simulink model "sgMdl_BMTS_FaultInsertionWithFIU"  (R2024b)
settings: Solver=FixedStepAuto  StartTime=0.0  StopTime=inf  RelTol=1e-3  EnableMultiTasking=on
undefined symbols (not defined in the file): Device_01, FIU12, FIU_12Ch_Set_init, sg_bce
libraries: slrealtimeethercatlib x27, simulink x13, SignalEditorBlockLib x1
Description:
  | BMTS - Fault Insertion with FIU
settings Model: ModifiedByFormat=Speedgoat  SimulationMode=external  ExtModeTrigDuration=100000  Creator=Speedgoat  LastModifiedBy=Speedgoat
settings SolverCC: ConcurrentTasks=on  AlgebraicLoopSolver=TrustRegion  PositivePriorityOrder=on  InsertRTBMode=Never (minimum delay)
settings DataIOCC: SaveFormat=Array  SaveState=on  SignalLoggingName=logsOut
settings OptimizationCC: BlockReduction=off  BooleanDataType=off  OptimizeBlockIOStorage=off  BufferReuse=off  ReuseModelBlockBuffer=off  GlobalBufferReuse=off  ExpressionFolding=off  LocalBlockOutputs=off  InitFltsAndDblsToZero=on  OptimizeDataStoreBuffers=off  BusAssignmentInplaceUpdate=off
settings DebuggingCC: SaveWithParameterizedLinksMsg=none  MergeDetectMultiDrivingBlocksExec=none  CheckExecutionContextPreStartOutputMsg=on  SignalResolutionControl=TryResolveAllWithWarning  TasksWithSamePriorityMsg=none  UnconnectedInputMsg=warning  UnconnectedOutputMsg=warning  UnconnectedLineMsg=warning  SFUnexpectedBacktrackingDiag=warning  SFNoUnconditionalDefaultTransitionDiag=warning  SFExecutionAtInitializationDiag=none  ArithmeticOperatorsInVariantConditions=warning
settings HardwareCC: ProdBitPerLong=64  ProdLongLongMode=on  ProdHWDeviceType=Intel->x86-64 (Linux 64)
settings ModelReferenceCC: EnableRefExpFcnMdlSchedulingChecks=on  PropagateSignalLabelsOutOfModel=off
settings SFSimCC: SimUseLocalCustomCode=off  SimTargetLang=C++
settings RTWCC: Description=Speedgoat Real-Time Target Machine  SystemTargetFile=speedgoat.tlc  TemplateMakefile=slrealtime_default_tmf  RTWUseLocalCustomCode=off  Toolchain=Simulink Real-Time Toolchain  BuildConfiguration=Faster Runs  TargetLang=C++  GPUComputeCapability=3.5  DLArmComputeVersion=19.05
settings CodeAppCC: StateflowObjectComments=on
settings SimulinkRealTimeTargetCC: SubcomponentCodeInterfacePackaging=Reusable function  InstructionSetFMA=off  LogToMDFFile=off  SLRTFileLogMaxRuns=10
settings ConfigComp: CovMetricSettings=dw  CovSaveCumulativeToWorkspaceVar=on  CovSaveSingleToWorkspaceVar=on  CovExternalEMLEnable=off  CovSFcnEnable=off  CovBoundaryAbsTol=1.0e-5

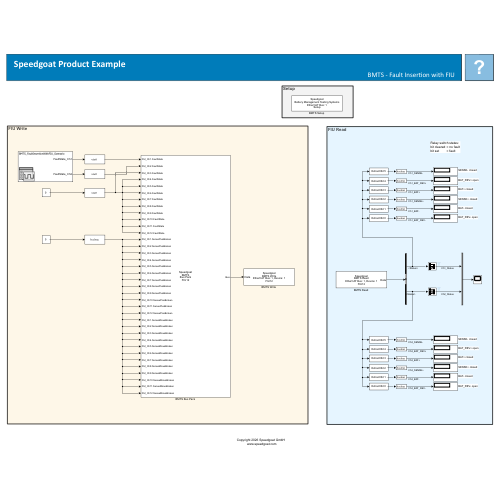
[thumbnail: Simulink's stored preview of the top-level diagram]
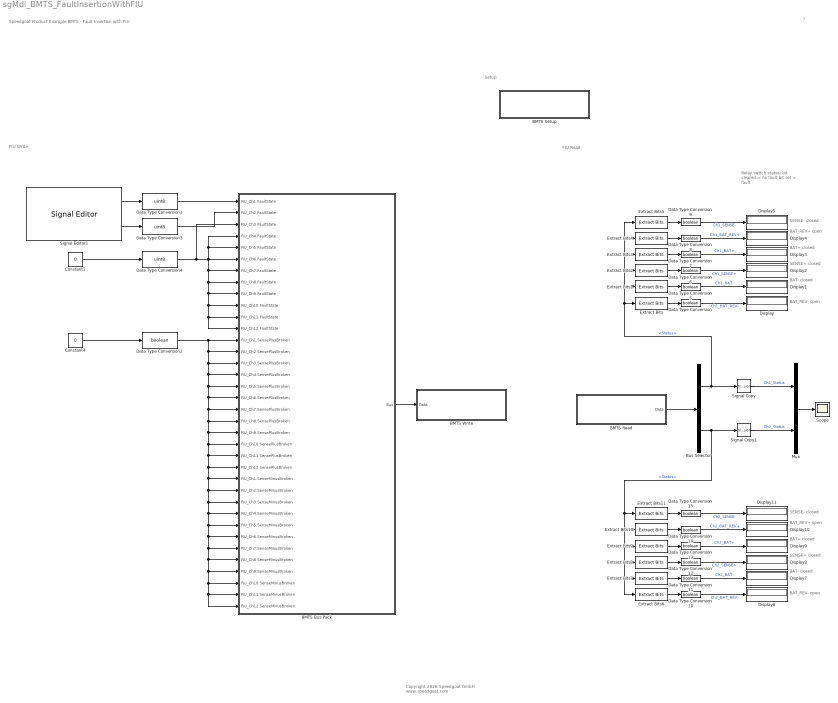
== system sgMdl_BMTS_FaultInsertionWithFIU ==
  note: BAT_REV- open
  note: Setup
  note: FIU Write
  note: FIU Read
  note: BAT- closed
  note: SENSE+ closed
  note: BAT+ closed
  note: BAT_REV+ open
  note: SENSE- closed
  note: Relay switch states:
      | bit cleared = no fault
      | bit set = fault
  note: BAT+ closed
  note: BAT_REV+ open
  note: BAT- closed
  note: SENSE+ closed
  note: BAT_REV- open
  note: SENSE- closed
  note: Speedgoat Product Example
      | BMTS - Fault Insertion with FIU
  note: ?
  note: Copyright 2026 Speedgoat GmbH
      |  www.speedgoat.com
  "BMTS Bus Pack " : Subsystem  mask(bmts_bus_pack){}
      settings: OpenFcn=sg_bce.openFcnBuspack;
      mask Help: eval('sg.utils.help.show(''io_main/refentry_bmts_buspack'');')
      mask Display: disp('Speedgoat\nBMTS\nBus Pack\nFIU12');
  "BMTS Read " : Subsystem  LoadFcn=sg_bce.createFiuTseBusSignals(12,0);  InitFcn=|  mask(bce_read){}
      | sg_bce.createFiuTseBusSignals(12,0);
      | sg_bce.checkNumberOfBlocksGlobal(bdroot);
      settings: OpenFcn=sg_bce.openFcnRead;
      mask Help: eval('sg.utils.help.show(''io_main/refentry_bce_read'');')
      mask Display: disp('Speedgoat\nBMTS Read\nEtherCAT Bus: 1, Device: 1\nFIU12');port_label('output',1,'Data');
  "BMTS Setup " : Subsystem  LoadFcn=|  InitFcn=|  mask(bce_setup){}
      LoadFcn=|
      | sg_bce.createBusSignals;
      | sg_bce.setupEniCallback(gcb, bdroot);
      InitFcn=|
      | sg_bce.createBusSignals;
      | sg_bce.checkNumberOfBlocksGlobal(bdroot);
      | sg_bce.setupEniCallback(gcb, bdroot);
      settings: OpenFcn=sg_bce.openFcnSetup;
      mask Help: eval('sg.utils.help.show(''io_main/refentry_bce_setup'');')
      mask Display: disp('Speedgoat\nBattery Management Testing Systems\nEtherCAT Bus: 1\nSetup');
  "BMTS Write " : Subsystem  LoadFcn=sg_bce.createFiuTseBusSignals(12,0);  InitFcn=|  mask(bce_write){}
      | sg_bce.createFiuTseBusSignals(12,0);
      | sg_bce.checkNumberOfBlocksGlobal(bdroot);
      settings: OpenFcn=sg_bce.openFcnWrite;
      mask Help: eval('sg.utils.help.show(''io_main/refentry_bce_write'');')
      mask Display: disp('Speedgoat\nBMTS Write\nEtherCAT Bus: 1, Device: 1\nFIU12');port_label('input',1,'Data');
  Bus Selector : BusSelector  OutputSignals=FIU_Ch1.Status,FIU_Ch2.Status
  Constant2 : Constant  Value=0
  Constant4 : Constant  Value=0
  Data Type Conversion{,2,5..15} (13 alike) : DataTypeConversion  OutDataTypeStr=boolean  SaturateOnIntegerOverflow=off  RndMeth=Floor
  Data Type Conversion1 : DataTypeConversion  OutDataTypeStr=uint8  SaturateOnIntegerOverflow=off  RndMeth=Floor
  Data Type Conversion3 : DataTypeConversion  OutDataTypeStr=uint8  SaturateOnIntegerOverflow=off  RndMeth=Floor
  Data Type Conversion4 : DataTypeConversion  OutDataTypeStr=uint8  SaturateOnIntegerOverflow=off  RndMeth=Floor
  Display{,1..11} (12 alike) : Display
  Extract Bits : simulink/Logic and Bit Operations/Extract Bits  bitsToExtract=Range of bits  numBits=8  bitIdxRange=[0]  outScalingMode=Treat bit field as an integer
  Extract Bits1 : simulink/Logic and Bit Operations/Extract Bits  bitsToExtract=Range of bits  numBits=8  bitIdxRange=[1]  outScalingMode=Treat bit field as an integer
  Extract Bits10 : simulink/Logic and Bit Operations/Extract Bits  bitsToExtract=Range of bits  numBits=8  bitIdxRange=[4]  outScalingMode=Treat bit field as an integer
  Extract Bits11 : simulink/Logic and Bit Operations/Extract Bits  bitsToExtract=Range of bits  numBits=8  bitIdxRange=[5]  outScalingMode=Treat bit field as an integer
  Extract Bits2 : simulink/Logic and Bit Operations/Extract Bits  bitsToExtract=Range of bits  numBits=8  bitIdxRange=[2]  outScalingMode=Treat bit field as an integer
  Extract Bits3 : simulink/Logic and Bit Operations/Extract Bits  bitsToExtract=Range of bits  numBits=8  bitIdxRange=[3]  outScalingMode=Treat bit field as an integer
  Extract Bits4 : simulink/Logic and Bit Operations/Extract Bits  bitsToExtract=Range of bits  numBits=8  bitIdxRange=[4]  outScalingMode=Treat bit field as an integer
  Extract Bits5 : simulink/Logic and Bit Operations/Extract Bits  bitsToExtract=Range of bits  numBits=8  bitIdxRange=[5]  outScalingMode=Treat bit field as an integer
  Extract Bits6 : simulink/Logic and Bit Operations/Extract Bits  bitsToExtract=Range of bits  numBits=8  bitIdxRange=[0]  outScalingMode=Treat bit field as an integer
  Extract Bits7 : simulink/Logic and Bit Operations/Extract Bits  bitsToExtract=Range of bits  numBits=8  bitIdxRange=[1]  outScalingMode=Treat bit field as an integer
  Extract Bits8 : simulink/Logic and Bit Operations/Extract Bits  bitsToExtract=Range of bits  numBits=8  bitIdxRange=[2]  outScalingMode=Treat bit field as an integer
  Extract Bits9 : simulink/Logic and Bit Operations/Extract Bits  bitsToExtract=Range of bits  numBits=8  bitIdxRange=[3]  outScalingMode=Treat bit field as an integer
  Mux : Mux  Inputs=2
  Scope : Scope
  Signal Copy : SignalConversion  OverrideOpt=off
  Signal Copy1 : SignalConversion  OverrideOpt=off
  Signal Editor1 : SignalEditorBlockLib/Signal Editor  FileName=BMTS_FaultInsertionWithFIU_Scenario.mat  ActiveScenario=BMTS_FaultInsertionWithFIU_Scenario  ActiveSignal=FaultState_Ch1  IsBus=off  OutputBusObjectStr=Bus: BusObject  SampleTime=0  Interpolate=off  ZeroCross=off  OutputAfterFinalValue=Setting to zero  Unit=inherit  PreserveSignalName=on  ApplySigPropsToAllScenarios=on  ApplySigPropsToAllSignals=off
  wires:
  "BMTS Read "/1(Data) -> Bus Selector/1
  Constant4/1 -> Data Type Conversion2/1
  Bus Selector/1 -> Extract Bits5/1, Extract Bits4/1, Extract Bits3/1, Extract Bits2/1, Extract Bits1/1, Extract Bits/1, Signal Copy/1  "<Status>"
  "BMTS Bus Pack "/1(Bus) -> "BMTS Write "/1(Data)
  Signal Editor1/1 -> Data Type Conversion1/1
  Data Type Conversion1/1 -> "BMTS Bus Pack "/1(FIU_Ch1.FaultState)
  Signal Editor1/2 -> Data Type Conversion3/1
  Data Type Conversion3/1 -> "BMTS Bus Pack "/2(FIU_Ch2.FaultState)
  Data Type Conversion2/1 -> "BMTS Bus Pack "/36(FIU_Ch12.SenseMinusBroken), "BMTS Bus Pack "/35(FIU_Ch11.SenseMinusBroken), "BMTS Bus Pack "/34(FIU_Ch10.SenseMinusBroken), "BMTS Bus Pack "/33(FIU_Ch9.SenseMinusBroken), "BMTS Bus Pack "/32(FIU_Ch8.SenseMinusBroken), "BMTS Bus Pack "/31(FIU_Ch7.SenseMinusBroken), "BMTS Bus Pack "/30(FIU_Ch6.SenseMinusBroken), "BMTS Bus Pack "/29(FIU_Ch5.SenseMinusBroken), "BMTS Bus Pack "/28(FIU_Ch4.SenseMinusBroken), "BMTS Bus Pack "/27(FIU_Ch3.SenseMinusBroken), "BMTS Bus Pack "/26(FIU_Ch2.SenseMinusBroken), "BMTS Bus Pack "/25(FIU_Ch1.SenseMinusBroken), "BMTS Bus Pack "/24(FIU_Ch12.SensePlusBroken), "BMTS Bus Pack "/23(FIU_Ch11.SensePlusBroken), "BMTS Bus Pack "/22(FIU_Ch10.SensePlusBroken), "BMTS Bus Pack "/21(FIU_Ch9.SensePlusBroken), "BMTS Bus Pack "/20(FIU_Ch8.SensePlusBroken), "BMTS Bus Pack "/19(FIU_Ch7.SensePlusBroken), "BMTS Bus Pack "/18(FIU_Ch6.SensePlusBroken), "BMTS Bus Pack "/17(FIU_Ch5.SensePlusBroken), "BMTS Bus Pack "/16(FIU_Ch4.SensePlusBroken), "BMTS Bus Pack "/15(FIU_Ch3.SensePlusBroken), "BMTS Bus Pack "/14(FIU_Ch2.SensePlusBroken), "BMTS Bus Pack "/13(FIU_Ch1.SensePlusBroken)
  Constant2/1 -> Data Type Conversion4/1
  Data Type Conversion4/1 -> "BMTS Bus Pack "/11(FIU_Ch11.FaultState), "BMTS Bus Pack "/12(FIU_Ch12.FaultState), "BMTS Bus Pack "/10(FIU_Ch10.FaultState), "BMTS Bus Pack "/9(FIU_Ch9.FaultState), "BMTS Bus Pack "/8(FIU_Ch8.FaultState), "BMTS Bus Pack "/7(FIU_Ch7.FaultState), "BMTS Bus Pack "/4(FIU_Ch4.FaultState), "BMTS Bus Pack "/5(FIU_Ch5.FaultState), "BMTS Bus Pack "/6(FIU_Ch6.FaultState), "BMTS Bus Pack "/3(FIU_Ch3.FaultState)
  Mux/1 -> Scope/1
  Extract Bits/1 -> Data Type Conversion/1
  Extract Bits1/1 -> Data Type Conversion5/1
  Extract Bits2/1 -> Data Type Conversion6/1
  Extract Bits5/1 -> Data Type Conversion9/1
  Extract Bits4/1 -> Data Type Conversion8/1
  Extract Bits3/1 -> Data Type Conversion7/1
  Extract Bits9/1 -> Data Type Conversion13/1
  Extract Bits10/1 -> Data Type Conversion14/1
  Extract Bits11/1 -> Data Type Conversion15/1
  Extract Bits8/1 -> Data Type Conversion12/1
  Extract Bits7/1 -> Data Type Conversion11/1
  Extract Bits6/1 -> Data Type Conversion10/1
  Bus Selector/2 -> Extract Bits6/1, Extract Bits7/1, Extract Bits8/1, Extract Bits9/1, Extract Bits10/1, Extract Bits11/1, Signal Copy1/1  "<Status>"
  Signal Copy/1 -> Mux/1  "Ch1_Status"
  Signal Copy1/1 -> Mux/2  "Ch2_Status"
  Data Type Conversion/1 -> Display/1  "Ch1_BAT_REV-"
  Data Type Conversion5/1 -> Display1/1  "Ch1_BAT-"
  Data Type Conversion6/1 -> Display2/1  "Ch1_SENSE+"
  Data Type Conversion7/1 -> Display3/1  "Ch1_BAT+"
  Data Type Conversion8/1 -> Display4/1  "Ch1_BAT_REV+"
  Data Type Conversion9/1 -> Display5/1  "Ch1_SENSE-"
  Data Type Conversion12/1 -> Display8/1  "Ch2_SENSE+"
  Data Type Conversion10/1 -> Display6/1  "Ch2_BAT_REV-"
  Data Type Conversion14/1 -> Display10/1  "Ch2_BAT_REV+"
  Data Type Conversion15/1 -> Display11/1  "Ch2_SENSE-"
  Data Type Conversion11/1 -> Display7/1  "Ch2_BAT-"
  Data Type Conversion13/1 -> Display9/1  "Ch2_BAT+"

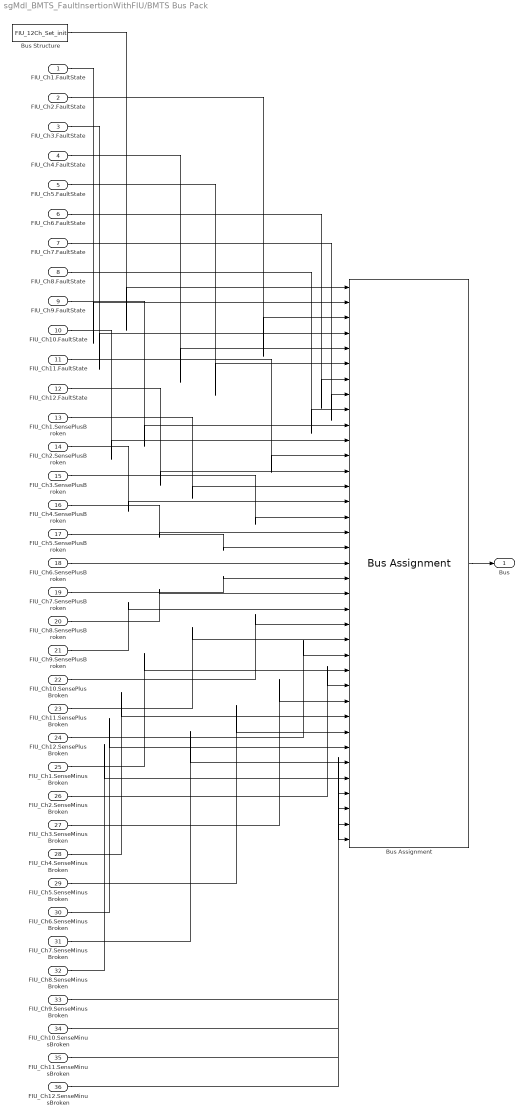
== system sgMdl_BMTS_FaultInsertionWithFIU/BMTS Bus Pack  ==
  FIU_Ch1.FaultState : Inport
  FIU_Ch2.FaultState : Inport  Port=2
  FIU_Ch3.FaultState : Inport  Port=3
  FIU_Ch4.FaultState : Inport  Port=4
  FIU_Ch5.FaultState : Inport  Port=5
  FIU_Ch6.FaultState : Inport  Port=6
  FIU_Ch7.FaultState : Inport  Port=7
  FIU_Ch8.FaultState : Inport  Port=8
  FIU_Ch9.FaultState : Inport  Port=9
  FIU_Ch10.FaultState : Inport  Port=10
  FIU_Ch11.FaultState : Inport  Port=11
  FIU_Ch12.FaultState : Inport  Port=12
  FIU_Ch1.SensePlusBroken : Inport  Port=13
  FIU_Ch2.SensePlusBroken : Inport  Port=14
  FIU_Ch3.SensePlusBroken : Inport  Port=15
  FIU_Ch4.SensePlusBroken : Inport  Port=16
  FIU_Ch5.SensePlusBroken : Inport  Port=17
  FIU_Ch6.SensePlusBroken : Inport  Port=18
  FIU_Ch7.SensePlusBroken : Inport  Port=19
  FIU_Ch8.SensePlusBroken : Inport  Port=20
  FIU_Ch9.SensePlusBroken : Inport  Port=21
  FIU_Ch10.SensePlusBroken : Inport  Port=22
  FIU_Ch11.SensePlusBroken : Inport  Port=23
  FIU_Ch12.SensePlusBroken : Inport  Port=24
  FIU_Ch1.SenseMinusBroken : Inport  Port=25
  FIU_Ch2.SenseMinusBroken : Inport  Port=26
  FIU_Ch3.SenseMinusBroken : Inport  Port=27
  FIU_Ch4.SenseMinusBroken : Inport  Port=28
  FIU_Ch5.SenseMinusBroken : Inport  Port=29
  FIU_Ch6.SenseMinusBroken : Inport  Port=30
  FIU_Ch7.SenseMinusBroken : Inport  Port=31
  FIU_Ch8.SenseMinusBroken : Inport  Port=32
  FIU_Ch9.SenseMinusBroken : Inport  Port=33
  FIU_Ch10.SenseMinusBroken : Inport  Port=34
  FIU_Ch11.SenseMinusBroken : Inport  Port=35
  FIU_Ch12.SenseMinusBroken : Inport  Port=36
  Bus Assignment : BusAssignment  AssignedSignals=FIU_Ch1.FaultState,FIU_Ch2.FaultState,FIU_Ch3.FaultState,FIU_Ch4.FaultState,FIU_Ch5.FaultState,FIU_Ch6.FaultState,FIU_Ch7.FaultState,FIU_Ch8.FaultState,FIU_Ch9.FaultState,FIU_Ch10.FaultState,FIU_Ch11.FaultState,FIU_Ch12.FaultState,FIU_Ch1.SensePlusBroken,FIU_Ch2.SensePlusBroken,FIU_Ch3.SensePlusBroken,FIU_Ch4.SensePlusBroken,FIU_Ch5.SensePlusBroken,FIU_Ch6.SensePlusBroken,FIU_Ch7.SensePlusBroken,FIU_Ch8.SensePlusBroken,FIU_Ch9.SensePlusBroken,FIU_Ch10.SensePlusBroken,FIU_Ch11.SensePlusBroken,FIU_Ch12.SensePlusBroken,FIU_Ch1.SenseMinusBroken,FIU_Ch2.SenseMinusBroken,FIU_Ch3.SenseMinusBroken,FIU_Ch4.SenseMinusBroken,FIU_Ch5.SenseMinusBroken,FIU_Ch6.SenseMinusBroken,FIU_Ch7.SenseMinusBroken,FIU_Ch8.SenseMinusBroken,FIU_Ch9.SenseMinusBroken,FIU_Ch10.SenseMinusBroken,FIU_Ch11.SenseMinusBroken,FIU_Ch12.SenseMinusBroken
  Bus Structure : Constant  Value=FIU_12Ch_Set_init  OutDataTypeStr=Bus: FIU_12Ch_Set
  Bus : Outport
  wires:
  Bus Structure/1 -> Bus Assignment/1
  FIU_Ch5.SenseMinusBroken/1 -> Bus Assignment/30
  FIU_Ch1.FaultState/1 -> Bus Assignment/2
  FIU_Ch2.FaultState/1 -> Bus Assignment/3
  FIU_Ch7.SenseMinusBroken/1 -> Bus Assignment/32
  FIU_Ch3.FaultState/1 -> Bus Assignment/4
  FIU_Ch5.FaultState/1 -> Bus Assignment/6
  FIU_Ch4.FaultState/1 -> Bus Assignment/5
  FIU_Ch2.SensePlusBroken/1 -> Bus Assignment/15
  FIU_Ch7.FaultState/1 -> Bus Assignment/8
  FIU_Ch8.SensePlusBroken/1 -> Bus Assignment/21
  FIU_Ch3.SensePlusBroken/1 -> Bus Assignment/16
  FIU_Ch8.FaultState/1 -> Bus Assignment/9
  FIU_Ch6.FaultState/1 -> Bus Assignment/7
  FIU_Ch7.SensePlusBroken/1 -> Bus Assignment/20
  FIU_Ch9.FaultState/1 -> Bus Assignment/10
  FIU_Ch10.FaultState/1 -> Bus Assignment/11
  FIU_Ch11.FaultState/1 -> Bus Assignment/12
  FIU_Ch12.FaultState/1 -> Bus Assignment/13
  FIU_Ch5.SensePlusBroken/1 -> Bus Assignment/18
  FIU_Ch1.SensePlusBroken/1 -> Bus Assignment/14
  FIU_Ch4.SensePlusBroken/1 -> Bus Assignment/17
  FIU_Ch2.SenseMinusBroken/1 -> Bus Assignment/27
  FIU_Ch6.SensePlusBroken/1 -> Bus Assignment/19
  FIU_Ch9.SensePlusBroken/1 -> Bus Assignment/22
  FIU_Ch10.SensePlusBroken/1 -> Bus Assignment/23
  FIU_Ch11.SensePlusBroken/1 -> Bus Assignment/24
  FIU_Ch12.SensePlusBroken/1 -> Bus Assignment/25
  FIU_Ch1.SenseMinusBroken/1 -> Bus Assignment/26
  FIU_Ch3.SenseMinusBroken/1 -> Bus Assignment/28
  FIU_Ch6.SenseMinusBroken/1 -> Bus Assignment/31
  FIU_Ch4.SenseMinusBroken/1 -> Bus Assignment/29
  FIU_Ch8.SenseMinusBroken/1 -> Bus Assignment/33
  FIU_Ch9.SenseMinusBroken/1 -> Bus Assignment/34
  FIU_Ch10.SenseMinusBroken/1 -> Bus Assignment/35
  FIU_Ch11.SenseMinusBroken/1 -> Bus Assignment/36
  FIU_Ch12.SenseMinusBroken/1 -> Bus Assignment/37
  Bus Assignment/1 -> Bus/1

== system sgMdl_BMTS_FaultInsertionWithFIU/BMTS Read  ==
  Subsystem : Subsystem
  Data : Outport  OutDataTypeStr=Bus: FIU_12Ch_Get
  wires:
  Subsystem/1(Data) -> Data/1

== system sgMdl_BMTS_FaultInsertionWithFIU/BMTS Setup  ==
  EtherCAT Init : slrealtimeethercatlib/EtherCAT Init  Priority=0  config_file=C:\Users\timo.straessle\AppData\Local\Temp\sg_bmts\sgMdl_BMTS_FaultInsertionWithFIU\sg_bmts_ENI_bus1.xml  device_id=1  portnum=1  initstate=2  dctuning=0  enaDebug=0  logFile='c:\dbglog.txt'  sample_time=0.001000  DCMode=0
  Terminator : Terminator
  wires:
  EtherCAT Init/1 -> Terminator/1

== system sgMdl_BMTS_FaultInsertionWithFIU/BMTS Write  ==
  Data : Inport  OutDataTypeStr=Bus: FIU_12Ch_Set
  Subsystem : Subsystem
  wires:
  Data/1 -> Subsystem/1(Data)

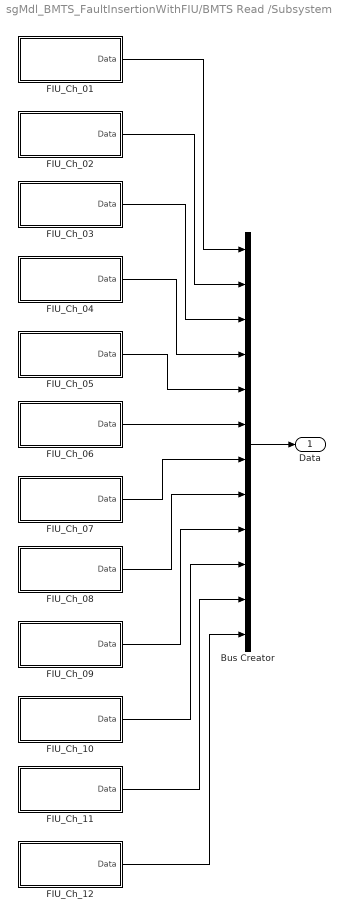
== system sgMdl_BMTS_FaultInsertionWithFIU/BMTS Read /Subsystem ==
  Bus Creator : BusCreator  Inputs=12  OutDataTypeStr=Bus: FIU_12Ch_Get
      settings: InheritFromInputs=off
  FIU_Ch_01 : Subsystem
  FIU_Ch_02 : Subsystem
  FIU_Ch_03 : Subsystem
  FIU_Ch_04 : Subsystem
  FIU_Ch_05 : Subsystem
  FIU_Ch_06 : Subsystem
  FIU_Ch_07 : Subsystem
  FIU_Ch_08 : Subsystem
  FIU_Ch_09 : Subsystem
  FIU_Ch_10 : Subsystem
  FIU_Ch_11 : Subsystem
  FIU_Ch_12 : Subsystem
  Data : Outport  OutDataTypeStr=Bus: FIU_12Ch_Get
  wires:
  FIU_Ch_05/1(Data) -> Bus Creator/5
  FIU_Ch_03/1(Data) -> Bus Creator/3
  FIU_Ch_01/1(Data) -> Bus Creator/1
  FIU_Ch_04/1(Data) -> Bus Creator/4
  FIU_Ch_02/1(Data) -> Bus Creator/2
  FIU_Ch_08/1(Data) -> Bus Creator/8
  FIU_Ch_06/1(Data) -> Bus Creator/6
  FIU_Ch_07/1(Data) -> Bus Creator/7
  FIU_Ch_09/1(Data) -> Bus Creator/9
  FIU_Ch_10/1(Data) -> Bus Creator/10
  FIU_Ch_11/1(Data) -> Bus Creator/11
  FIU_Ch_12/1(Data) -> Bus Creator/12
  Bus Creator/1 -> Data/1

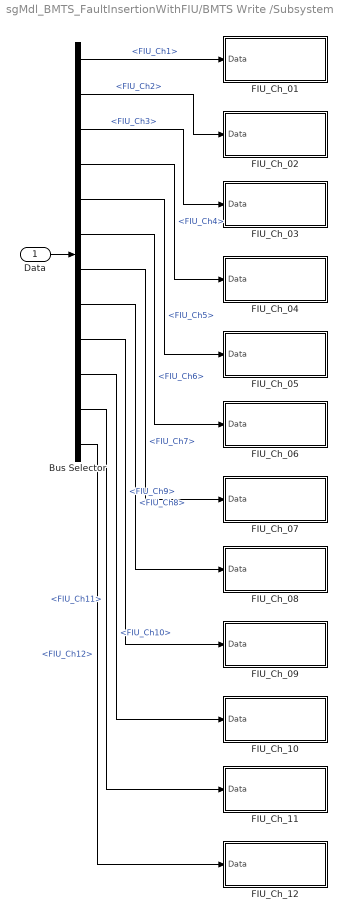
== system sgMdl_BMTS_FaultInsertionWithFIU/BMTS Write /Subsystem ==
  Data : Inport  OutDataTypeStr=Bus: FIU_12Ch_Set
  Bus Selector : BusSelector  OutputSignals=FIU_Ch1,FIU_Ch2,FIU_Ch3,FIU_Ch4,FIU_Ch5,FIU_Ch6,FIU_Ch7,FIU_Ch8,FIU_Ch9,FIU_Ch10,FIU_Ch11,FIU_Ch12
  FIU_Ch_01 : Subsystem
  FIU_Ch_02 : Subsystem
  FIU_Ch_03 : Subsystem
  FIU_Ch_04 : Subsystem
  FIU_Ch_05 : Subsystem
  FIU_Ch_06 : Subsystem
  FIU_Ch_07 : Subsystem
  FIU_Ch_08 : Subsystem
  FIU_Ch_09 : Subsystem
  FIU_Ch_10 : Subsystem
  FIU_Ch_11 : Subsystem
  FIU_Ch_12 : Subsystem
  wires:
  Data/1 -> Bus Selector/1
  Bus Selector/7 -> FIU_Ch_07/1(Data)  "<FIU_Ch7>"
  Bus Selector/6 -> FIU_Ch_06/1(Data)  "<FIU_Ch6>"
  Bus Selector/4 -> FIU_Ch_04/1(Data)  "<FIU_Ch4>"
  Bus Selector/3 -> FIU_Ch_03/1(Data)  "<FIU_Ch3>"
  Bus Selector/2 -> FIU_Ch_02/1(Data)  "<FIU_Ch2>"
  Bus Selector/1 -> FIU_Ch_01/1(Data)  "<FIU_Ch1>"
  Bus Selector/5 -> FIU_Ch_05/1(Data)  "<FIU_Ch5>"
  Bus Selector/8 -> FIU_Ch_08/1(Data)  "<FIU_Ch8>"
  Bus Selector/9 -> FIU_Ch_09/1(Data)  "<FIU_Ch9>"
  Bus Selector/10 -> FIU_Ch_10/1(Data)  "<FIU_Ch10>"
  Bus Selector/11 -> FIU_Ch_11/1(Data)  "<FIU_Ch11>"
  Bus Selector/12 -> FIU_Ch_12/1(Data)  "<FIU_Ch12>"

== system sgMdl_BMTS_FaultInsertionWithFIU/BMTS Read /Subsystem/FIU_Ch_01 ==
  note: Channel X
  Bus Creator : BusCreator  Inputs=1  OutDataTypeStr=Bus: FIU_Get
      settings: InheritFromInputs=off
  EtherCAT PDO Receive01 : slrealtimeethercatlib/EtherCAT PDO Receive  Priority=2  sig_name=Device_01 (FIU12).Tx_Channel_01.status  sig_offset=0  sig_type=uint8  type_size=8  sig_dim=1  device_id=1  sample_time=0.001000
  Data : Outport  OutDataTypeStr=Bus: FIU_Get
  wires:
  Bus Creator/1 -> Data/1
  EtherCAT PDO Receive01/1 -> Bus Creator/1  "ChX_Status"

== system sgMdl_BMTS_FaultInsertionWithFIU/BMTS Read /Subsystem/FIU_Ch_02 ==
  note: Channel X
  Bus Creator : BusCreator  Inputs=1  OutDataTypeStr=Bus: FIU_Get
      settings: InheritFromInputs=off
  EtherCAT PDO Receive01 : slrealtimeethercatlib/EtherCAT PDO Receive  Priority=2  sig_name=Device_01 (FIU12).Tx_Channel_02.status  sig_offset=8  sig_type=uint8  type_size=8  sig_dim=1  device_id=1  sample_time=0.001000
  Data : Outport  OutDataTypeStr=Bus: FIU_Get
  wires:
  Bus Creator/1 -> Data/1
  EtherCAT PDO Receive01/1 -> Bus Creator/1  "ChX_Status"

== system sgMdl_BMTS_FaultInsertionWithFIU/BMTS Read /Subsystem/FIU_Ch_03 ==
  note: Channel X
  Bus Creator : BusCreator  Inputs=1  OutDataTypeStr=Bus: FIU_Get
      settings: InheritFromInputs=off
  EtherCAT PDO Receive01 : slrealtimeethercatlib/EtherCAT PDO Receive  Priority=2  sig_name=Device_01 (FIU12).Tx_Channel_03.status  sig_offset=16  sig_type=uint8  type_size=8  sig_dim=1  device_id=1  sample_time=0.001000
  Data : Outport  OutDataTypeStr=Bus: FIU_Get
  wires:
  Bus Creator/1 -> Data/1
  EtherCAT PDO Receive01/1 -> Bus Creator/1  "ChX_Status"

== system sgMdl_BMTS_FaultInsertionWithFIU/BMTS Read /Subsystem/FIU_Ch_04 ==
  note: Channel X
  Bus Creator : BusCreator  Inputs=1  OutDataTypeStr=Bus: FIU_Get
      settings: InheritFromInputs=off
  EtherCAT PDO Receive01 : slrealtimeethercatlib/EtherCAT PDO Receive  Priority=2  sig_name=Device_01 (FIU12).Tx_Channel_04.status  sig_offset=24  sig_type=uint8  type_size=8  sig_dim=1  device_id=1  sample_time=0.001000
  Data : Outport  OutDataTypeStr=Bus: FIU_Get
  wires:
  Bus Creator/1 -> Data/1
  EtherCAT PDO Receive01/1 -> Bus Creator/1  "ChX_Status"

== system sgMdl_BMTS_FaultInsertionWithFIU/BMTS Read /Subsystem/FIU_Ch_05 ==
  note: Channel X
  Bus Creator : BusCreator  Inputs=1  OutDataTypeStr=Bus: FIU_Get
      settings: InheritFromInputs=off
  EtherCAT PDO Receive01 : slrealtimeethercatlib/EtherCAT PDO Receive  Priority=2  sig_name=Device_01 (FIU12).Tx_Channel_05.status  sig_offset=32  sig_type=uint8  type_size=8  sig_dim=1  device_id=1  sample_time=0.001000
  Data : Outport  OutDataTypeStr=Bus: FIU_Get
  wires:
  Bus Creator/1 -> Data/1
  EtherCAT PDO Receive01/1 -> Bus Creator/1  "ChX_Status"

== system sgMdl_BMTS_FaultInsertionWithFIU/BMTS Read /Subsystem/FIU_Ch_06 ==
  note: Channel X
  Bus Creator : BusCreator  Inputs=1  OutDataTypeStr=Bus: FIU_Get
      settings: InheritFromInputs=off
  EtherCAT PDO Receive01 : slrealtimeethercatlib/EtherCAT PDO Receive  Priority=2  sig_name=Device_01 (FIU12).Tx_Channel_06.status  sig_offset=40  sig_type=uint8  type_size=8  sig_dim=1  device_id=1  sample_time=0.001000
  Data : Outport  OutDataTypeStr=Bus: FIU_Get
  wires:
  Bus Creator/1 -> Data/1
  EtherCAT PDO Receive01/1 -> Bus Creator/1  "ChX_Status"

== system sgMdl_BMTS_FaultInsertionWithFIU/BMTS Read /Subsystem/FIU_Ch_07 ==
  note: Channel X
  Bus Creator : BusCreator  Inputs=1  OutDataTypeStr=Bus: FIU_Get
      settings: InheritFromInputs=off
  EtherCAT PDO Receive01 : slrealtimeethercatlib/EtherCAT PDO Receive  Priority=2  sig_name=Device_01 (FIU12).Tx_Channel_07.status  sig_offset=48  sig_type=uint8  type_size=8  sig_dim=1  device_id=1  sample_time=0.001000
  Data : Outport  OutDataTypeStr=Bus: FIU_Get
  wires:
  Bus Creator/1 -> Data/1
  EtherCAT PDO Receive01/1 -> Bus Creator/1  "ChX_Status"

== system sgMdl_BMTS_FaultInsertionWithFIU/BMTS Read /Subsystem/FIU_Ch_08 ==
  note: Channel X
  Bus Creator : BusCreator  Inputs=1  OutDataTypeStr=Bus: FIU_Get
      settings: InheritFromInputs=off
  EtherCAT PDO Receive01 : slrealtimeethercatlib/EtherCAT PDO Receive  Priority=2  sig_name=Device_01 (FIU12).Tx_Channel_08.status  sig_offset=56  sig_type=uint8  type_size=8  sig_dim=1  device_id=1  sample_time=0.001000
  Data : Outport  OutDataTypeStr=Bus: FIU_Get
  wires:
  Bus Creator/1 -> Data/1
  EtherCAT PDO Receive01/1 -> Bus Creator/1  "ChX_Status"

== system sgMdl_BMTS_FaultInsertionWithFIU/BMTS Read /Subsystem/FIU_Ch_09 ==
  note: Channel X
  Bus Creator : BusCreator  Inputs=1  OutDataTypeStr=Bus: FIU_Get
      settings: InheritFromInputs=off
  EtherCAT PDO Receive01 : slrealtimeethercatlib/EtherCAT PDO Receive  Priority=2  sig_name=Device_01 (FIU12).Tx_Channel_09.status  sig_offset=64  sig_type=uint8  type_size=8  sig_dim=1  device_id=1  sample_time=0.001000
  Data : Outport  OutDataTypeStr=Bus: FIU_Get
  wires:
  Bus Creator/1 -> Data/1
  EtherCAT PDO Receive01/1 -> Bus Creator/1  "ChX_Status"

== system sgMdl_BMTS_FaultInsertionWithFIU/BMTS Read /Subsystem/FIU_Ch_10 ==
  note: Channel X
  Bus Creator : BusCreator  Inputs=1  OutDataTypeStr=Bus: FIU_Get
      settings: InheritFromInputs=off
  EtherCAT PDO Receive01 : slrealtimeethercatlib/EtherCAT PDO Receive  Priority=2  sig_name=Device_01 (FIU12).Tx_Channel_10.status  sig_offset=72  sig_type=uint8  type_size=8  sig_dim=1  device_id=1  sample_time=0.001000
  Data : Outport  OutDataTypeStr=Bus: FIU_Get
  wires:
  Bus Creator/1 -> Data/1
  EtherCAT PDO Receive01/1 -> Bus Creator/1  "ChX_Status"

== system sgMdl_BMTS_FaultInsertionWithFIU/BMTS Read /Subsystem/FIU_Ch_11 ==
  note: Channel X
  Bus Creator : BusCreator  Inputs=1  OutDataTypeStr=Bus: FIU_Get
      settings: InheritFromInputs=off
  EtherCAT PDO Receive01 : slrealtimeethercatlib/EtherCAT PDO Receive  Priority=2  sig_name=Device_01 (FIU12).Tx_Channel_11.status  sig_offset=80  sig_type=uint8  type_size=8  sig_dim=1  device_id=1  sample_time=0.001000
  Data : Outport  OutDataTypeStr=Bus: FIU_Get
  wires:
  Bus Creator/1 -> Data/1
  EtherCAT PDO Receive01/1 -> Bus Creator/1  "ChX_Status"

== system sgMdl_BMTS_FaultInsertionWithFIU/BMTS Read /Subsystem/FIU_Ch_12 ==
  note: Channel X
  Bus Creator : BusCreator  Inputs=1  OutDataTypeStr=Bus: FIU_Get
      settings: InheritFromInputs=off
  EtherCAT PDO Receive01 : slrealtimeethercatlib/EtherCAT PDO Receive  Priority=2  sig_name=Device_01 (FIU12).Tx_Channel_12.status  sig_offset=88  sig_type=uint8  type_size=8  sig_dim=1  device_id=1  sample_time=0.001000
  Data : Outport  OutDataTypeStr=Bus: FIU_Get
  wires:
  Bus Creator/1 -> Data/1
  EtherCAT PDO Receive01/1 -> Bus Creator/1  "ChX_Status"

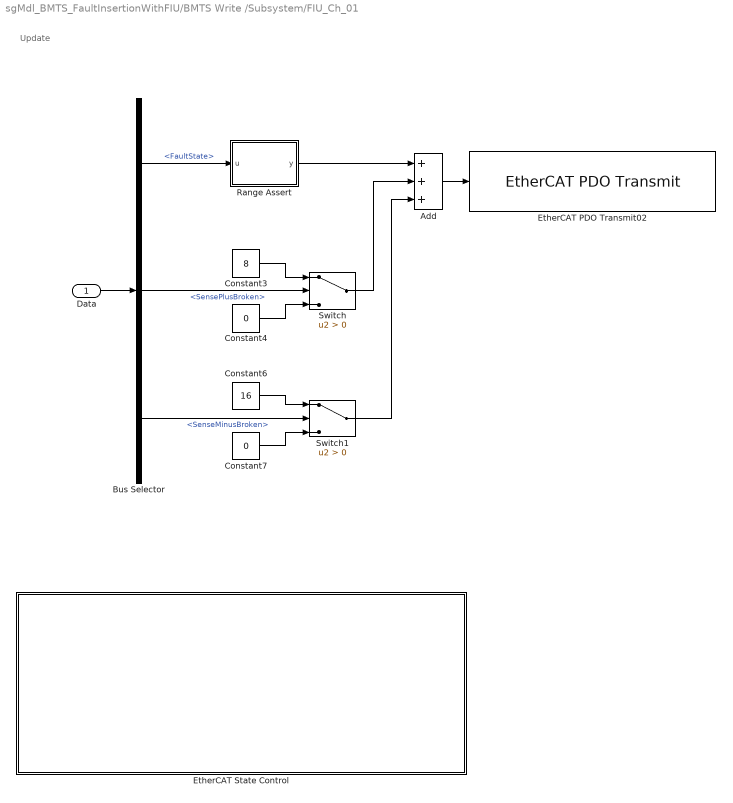
== system sgMdl_BMTS_FaultInsertionWithFIU/BMTS Write /Subsystem/FIU_Ch_01 ==
  note: Update
  Data : Inport  OutDataTypeStr=Bus: FIU_Set
  Add : Sum  Inputs=+++
  Bus Selector : BusSelector  OutputSignals=FaultState,SensePlusBroken,SenseMinusBroken
  Constant3 : Constant  Value=8  OutDataTypeStr=uint8
  Constant4 : Constant  Value=0  OutDataTypeStr=uint8
  Constant6 : Constant  Value=16  OutDataTypeStr=uint8
  Constant7 : Constant  Value=0  OutDataTypeStr=uint8
  EtherCAT PDO Transmit02 : slrealtimeethercatlib/EtherCAT PDO Transmit  Priority=3  sig_name=Device_01 (FIU12).Rx_Channel_01.faultState  sig_offset=0  sig_type=uint8  type_size=8  sig_dim=1  device_id=1  sample_time=0.001000
  EtherCAT State Control : Subsystem
  Range Assert : MATLAB Function  TreatAsAtomicUnit=on
  Switch : Switch  Criteria=u2 > Threshold  SaturateOnIntegerOverflow=off  InputSameDT=off
  Switch1 : Switch  Criteria=u2 > Threshold  SaturateOnIntegerOverflow=off  InputSameDT=off
  wires:
  Range Assert/1(y) -> Add/1
  Data/1 -> Bus Selector/1
  Bus Selector/2 -> Switch/2  "<SensePlusBroken>"
  Constant6/1 -> Switch1/1
  Constant3/1 -> Switch/1
  Switch/1 -> Add/2
  Constant4/1 -> Switch/3
  Constant7/1 -> Switch1/3
  Add/1 -> EtherCAT PDO Transmit02/1
  Bus Selector/3 -> Switch1/2  "<SenseMinusBroken>"
  Switch1/1 -> Add/3
  Bus Selector/1 -> Range Assert/1(u)  "<FaultState>"

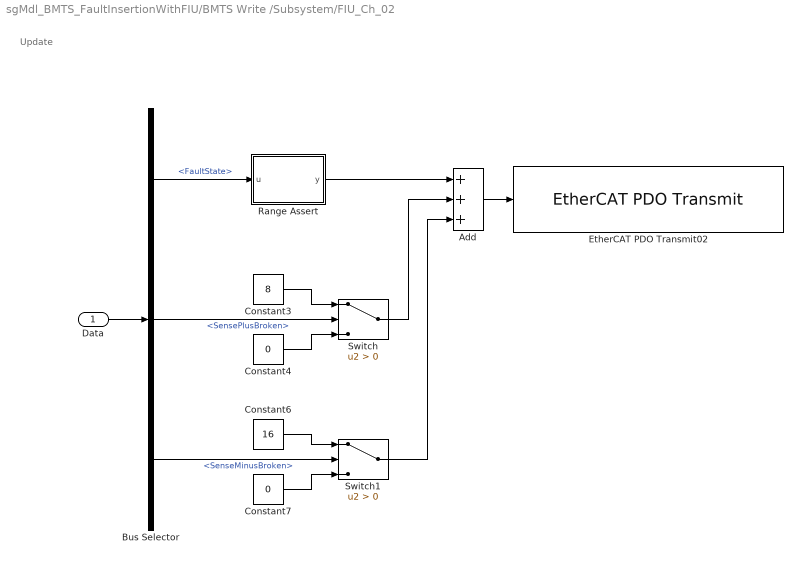
== system sgMdl_BMTS_FaultInsertionWithFIU/BMTS Write /Subsystem/FIU_Ch_02 ==
  note: Update
  Data : Inport  OutDataTypeStr=Bus: FIU_Set
  Add : Sum  Inputs=+++
  Bus Selector : BusSelector  OutputSignals=FaultState,SensePlusBroken,SenseMinusBroken
  Constant3 : Constant  Value=8  OutDataTypeStr=uint8
  Constant4 : Constant  Value=0  OutDataTypeStr=uint8
  Constant6 : Constant  Value=16  OutDataTypeStr=uint8
  Constant7 : Constant  Value=0  OutDataTypeStr=uint8
  EtherCAT PDO Transmit02 : slrealtimeethercatlib/EtherCAT PDO Transmit  Priority=3  sig_name=Device_01 (FIU12).Rx_Channel_02.faultState  sig_offset=8  sig_type=uint8  type_size=8  sig_dim=1  device_id=1  sample_time=0.001000
  Range Assert : MATLAB Function  TreatAsAtomicUnit=on
  Switch : Switch  Criteria=u2 > Threshold  SaturateOnIntegerOverflow=off  InputSameDT=off
  Switch1 : Switch  Criteria=u2 > Threshold  SaturateOnIntegerOverflow=off  InputSameDT=off
  wires:
  Range Assert/1(y) -> Add/1
  Data/1 -> Bus Selector/1
  Bus Selector/2 -> Switch/2  "<SensePlusBroken>"
  Constant6/1 -> Switch1/1
  Constant3/1 -> Switch/1
  Switch/1 -> Add/2
  Constant4/1 -> Switch/3
  Constant7/1 -> Switch1/3
  Add/1 -> EtherCAT PDO Transmit02/1
  Bus Selector/3 -> Switch1/2  "<SenseMinusBroken>"
  Switch1/1 -> Add/3
  Bus Selector/1 -> Range Assert/1(u)  "<FaultState>"

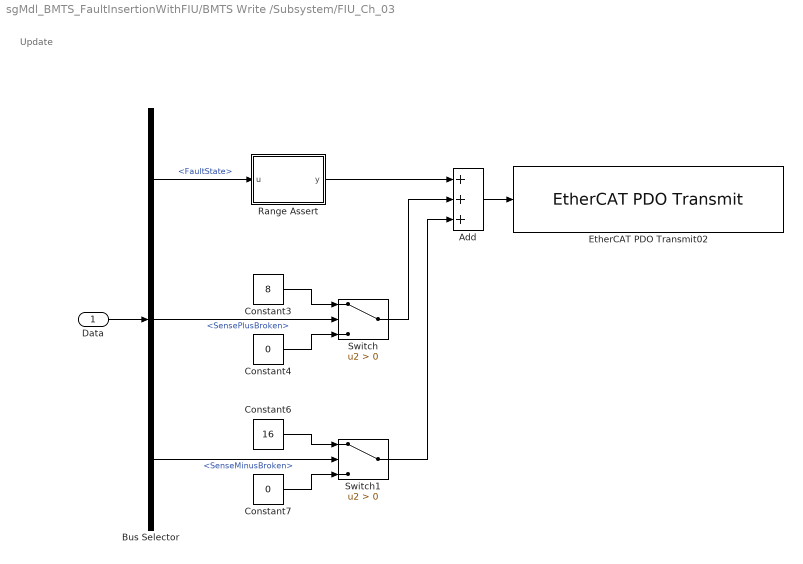
== system sgMdl_BMTS_FaultInsertionWithFIU/BMTS Write /Subsystem/FIU_Ch_03 ==
  note: Update
  Data : Inport  OutDataTypeStr=Bus: FIU_Set
  Add : Sum  Inputs=+++
  Bus Selector : BusSelector  OutputSignals=FaultState,SensePlusBroken,SenseMinusBroken
  Constant3 : Constant  Value=8  OutDataTypeStr=uint8
  Constant4 : Constant  Value=0  OutDataTypeStr=uint8
  Constant6 : Constant  Value=16  OutDataTypeStr=uint8
  Constant7 : Constant  Value=0  OutDataTypeStr=uint8
  EtherCAT PDO Transmit02 : slrealtimeethercatlib/EtherCAT PDO Transmit  Priority=3  sig_name=Device_01 (FIU12).Rx_Channel_03.faultState  sig_offset=16  sig_type=uint8  type_size=8  sig_dim=1  device_id=1  sample_time=0.001000
  Range Assert : MATLAB Function  TreatAsAtomicUnit=on
  Switch : Switch  Criteria=u2 > Threshold  SaturateOnIntegerOverflow=off  InputSameDT=off
  Switch1 : Switch  Criteria=u2 > Threshold  SaturateOnIntegerOverflow=off  InputSameDT=off
  wires:
  Range Assert/1(y) -> Add/1
  Data/1 -> Bus Selector/1
  Bus Selector/2 -> Switch/2  "<SensePlusBroken>"
  Constant6/1 -> Switch1/1
  Constant3/1 -> Switch/1
  Switch/1 -> Add/2
  Constant4/1 -> Switch/3
  Constant7/1 -> Switch1/3
  Add/1 -> EtherCAT PDO Transmit02/1
  Bus Selector/3 -> Switch1/2  "<SenseMinusBroken>"
  Switch1/1 -> Add/3
  Bus Selector/1 -> Range Assert/1(u)  "<FaultState>"

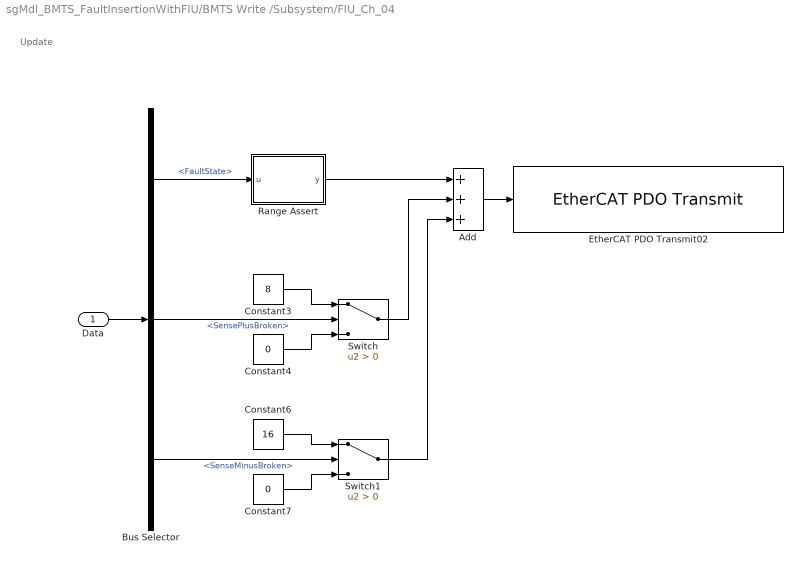
== system sgMdl_BMTS_FaultInsertionWithFIU/BMTS Write /Subsystem/FIU_Ch_04 ==
  note: Update
  Data : Inport  OutDataTypeStr=Bus: FIU_Set
  Add : Sum  Inputs=+++
  Bus Selector : BusSelector  OutputSignals=FaultState,SensePlusBroken,SenseMinusBroken
  Constant3 : Constant  Value=8  OutDataTypeStr=uint8
  Constant4 : Constant  Value=0  OutDataTypeStr=uint8
  Constant6 : Constant  Value=16  OutDataTypeStr=uint8
  Constant7 : Constant  Value=0  OutDataTypeStr=uint8
  EtherCAT PDO Transmit02 : slrealtimeethercatlib/EtherCAT PDO Transmit  Priority=3  sig_name=Device_01 (FIU12).Rx_Channel_04.faultState  sig_offset=24  sig_type=uint8  type_size=8  sig_dim=1  device_id=1  sample_time=0.001000
  Range Assert : MATLAB Function  TreatAsAtomicUnit=on
  Switch : Switch  Criteria=u2 > Threshold  SaturateOnIntegerOverflow=off  InputSameDT=off
  Switch1 : Switch  Criteria=u2 > Threshold  SaturateOnIntegerOverflow=off  InputSameDT=off
  wires:
  Range Assert/1(y) -> Add/1
  Data/1 -> Bus Selector/1
  Bus Selector/2 -> Switch/2  "<SensePlusBroken>"
  Constant6/1 -> Switch1/1
  Constant3/1 -> Switch/1
  Switch/1 -> Add/2
  Constant4/1 -> Switch/3
  Constant7/1 -> Switch1/3
  Add/1 -> EtherCAT PDO Transmit02/1
  Bus Selector/3 -> Switch1/2  "<SenseMinusBroken>"
  Switch1/1 -> Add/3
  Bus Selector/1 -> Range Assert/1(u)  "<FaultState>"

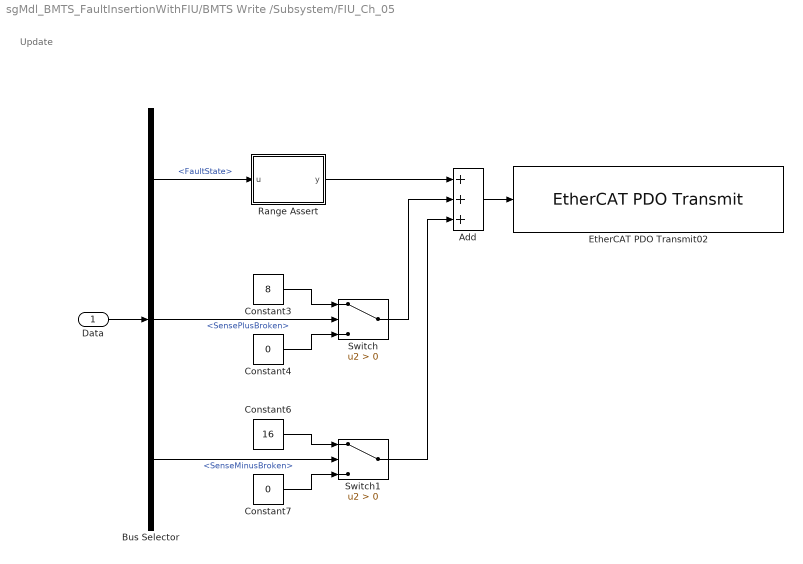
== system sgMdl_BMTS_FaultInsertionWithFIU/BMTS Write /Subsystem/FIU_Ch_05 ==
  note: Update
  Data : Inport  OutDataTypeStr=Bus: FIU_Set
  Add : Sum  Inputs=+++
  Bus Selector : BusSelector  OutputSignals=FaultState,SensePlusBroken,SenseMinusBroken
  Constant3 : Constant  Value=8  OutDataTypeStr=uint8
  Constant4 : Constant  Value=0  OutDataTypeStr=uint8
  Constant6 : Constant  Value=16  OutDataTypeStr=uint8
  Constant7 : Constant  Value=0  OutDataTypeStr=uint8
  EtherCAT PDO Transmit02 : slrealtimeethercatlib/EtherCAT PDO Transmit  Priority=3  sig_name=Device_01 (FIU12).Rx_Channel_05.faultState  sig_offset=32  sig_type=uint8  type_size=8  sig_dim=1  device_id=1  sample_time=0.001000
  Range Assert : MATLAB Function  TreatAsAtomicUnit=on
  Switch : Switch  Criteria=u2 > Threshold  SaturateOnIntegerOverflow=off  InputSameDT=off
  Switch1 : Switch  Criteria=u2 > Threshold  SaturateOnIntegerOverflow=off  InputSameDT=off
  wires:
  Range Assert/1(y) -> Add/1
  Data/1 -> Bus Selector/1
  Bus Selector/2 -> Switch/2  "<SensePlusBroken>"
  Constant6/1 -> Switch1/1
  Constant3/1 -> Switch/1
  Switch/1 -> Add/2
  Constant4/1 -> Switch/3
  Constant7/1 -> Switch1/3
  Add/1 -> EtherCAT PDO Transmit02/1
  Bus Selector/3 -> Switch1/2  "<SenseMinusBroken>"
  Switch1/1 -> Add/3
  Bus Selector/1 -> Range Assert/1(u)  "<FaultState>"

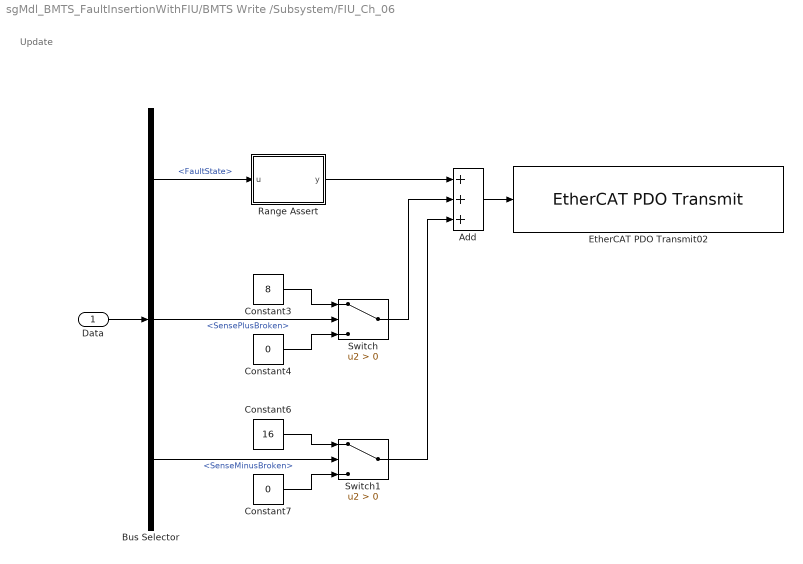
== system sgMdl_BMTS_FaultInsertionWithFIU/BMTS Write /Subsystem/FIU_Ch_06 ==
  note: Update
  Data : Inport  OutDataTypeStr=Bus: FIU_Set
  Add : Sum  Inputs=+++
  Bus Selector : BusSelector  OutputSignals=FaultState,SensePlusBroken,SenseMinusBroken
  Constant3 : Constant  Value=8  OutDataTypeStr=uint8
  Constant4 : Constant  Value=0  OutDataTypeStr=uint8
  Constant6 : Constant  Value=16  OutDataTypeStr=uint8
  Constant7 : Constant  Value=0  OutDataTypeStr=uint8
  EtherCAT PDO Transmit02 : slrealtimeethercatlib/EtherCAT PDO Transmit  Priority=3  sig_name=Device_01 (FIU12).Rx_Channel_06.faultState  sig_offset=40  sig_type=uint8  type_size=8  sig_dim=1  device_id=1  sample_time=0.001000
  Range Assert : MATLAB Function  TreatAsAtomicUnit=on
  Switch : Switch  Criteria=u2 > Threshold  SaturateOnIntegerOverflow=off  InputSameDT=off
  Switch1 : Switch  Criteria=u2 > Threshold  SaturateOnIntegerOverflow=off  InputSameDT=off
  wires:
  Range Assert/1(y) -> Add/1
  Data/1 -> Bus Selector/1
  Bus Selector/2 -> Switch/2  "<SensePlusBroken>"
  Constant6/1 -> Switch1/1
  Constant3/1 -> Switch/1
  Switch/1 -> Add/2
  Constant4/1 -> Switch/3
  Constant7/1 -> Switch1/3
  Add/1 -> EtherCAT PDO Transmit02/1
  Bus Selector/3 -> Switch1/2  "<SenseMinusBroken>"
  Switch1/1 -> Add/3
  Bus Selector/1 -> Range Assert/1(u)  "<FaultState>"

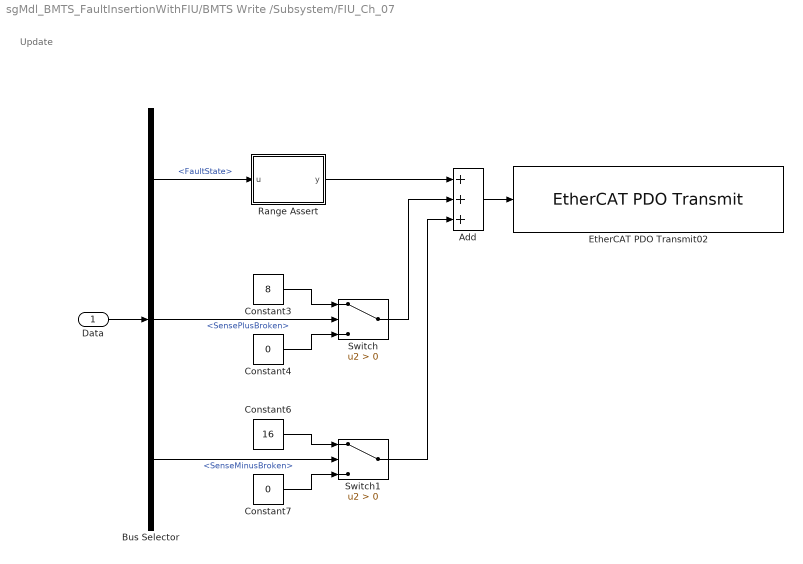
== system sgMdl_BMTS_FaultInsertionWithFIU/BMTS Write /Subsystem/FIU_Ch_07 ==
  note: Update
  Data : Inport  OutDataTypeStr=Bus: FIU_Set
  Add : Sum  Inputs=+++
  Bus Selector : BusSelector  OutputSignals=FaultState,SensePlusBroken,SenseMinusBroken
  Constant3 : Constant  Value=8  OutDataTypeStr=uint8
  Constant4 : Constant  Value=0  OutDataTypeStr=uint8
  Constant6 : Constant  Value=16  OutDataTypeStr=uint8
  Constant7 : Constant  Value=0  OutDataTypeStr=uint8
  EtherCAT PDO Transmit02 : slrealtimeethercatlib/EtherCAT PDO Transmit  Priority=3  sig_name=Device_01 (FIU12).Rx_Channel_07.faultState  sig_offset=48  sig_type=uint8  type_size=8  sig_dim=1  device_id=1  sample_time=0.001000
  Range Assert : MATLAB Function  TreatAsAtomicUnit=on
  Switch : Switch  Criteria=u2 > Threshold  SaturateOnIntegerOverflow=off  InputSameDT=off
  Switch1 : Switch  Criteria=u2 > Threshold  SaturateOnIntegerOverflow=off  InputSameDT=off
  wires:
  Range Assert/1(y) -> Add/1
  Data/1 -> Bus Selector/1
  Bus Selector/2 -> Switch/2  "<SensePlusBroken>"
  Constant6/1 -> Switch1/1
  Constant3/1 -> Switch/1
  Switch/1 -> Add/2
  Constant4/1 -> Switch/3
  Constant7/1 -> Switch1/3
  Add/1 -> EtherCAT PDO Transmit02/1
  Bus Selector/3 -> Switch1/2  "<SenseMinusBroken>"
  Switch1/1 -> Add/3
  Bus Selector/1 -> Range Assert/1(u)  "<FaultState>"

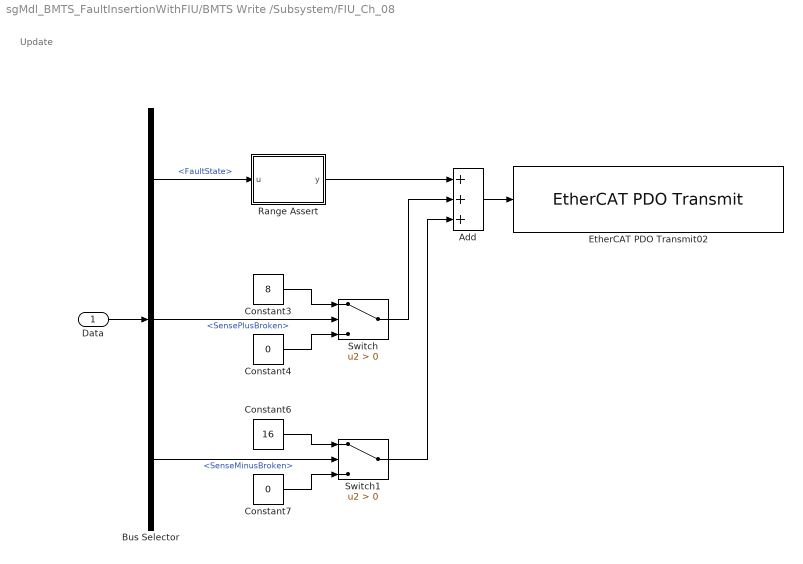
== system sgMdl_BMTS_FaultInsertionWithFIU/BMTS Write /Subsystem/FIU_Ch_08 ==
  note: Update
  Data : Inport  OutDataTypeStr=Bus: FIU_Set
  Add : Sum  Inputs=+++
  Bus Selector : BusSelector  OutputSignals=FaultState,SensePlusBroken,SenseMinusBroken
  Constant3 : Constant  Value=8  OutDataTypeStr=uint8
  Constant4 : Constant  Value=0  OutDataTypeStr=uint8
  Constant6 : Constant  Value=16  OutDataTypeStr=uint8
  Constant7 : Constant  Value=0  OutDataTypeStr=uint8
  EtherCAT PDO Transmit02 : slrealtimeethercatlib/EtherCAT PDO Transmit  Priority=3  sig_name=Device_01 (FIU12).Rx_Channel_08.faultState  sig_offset=56  sig_type=uint8  type_size=8  sig_dim=1  device_id=1  sample_time=0.001000
  Range Assert : MATLAB Function  TreatAsAtomicUnit=on
  Switch : Switch  Criteria=u2 > Threshold  SaturateOnIntegerOverflow=off  InputSameDT=off
  Switch1 : Switch  Criteria=u2 > Threshold  SaturateOnIntegerOverflow=off  InputSameDT=off
  wires:
  Range Assert/1(y) -> Add/1
  Data/1 -> Bus Selector/1
  Bus Selector/2 -> Switch/2  "<SensePlusBroken>"
  Constant6/1 -> Switch1/1
  Constant3/1 -> Switch/1
  Switch/1 -> Add/2
  Constant4/1 -> Switch/3
  Constant7/1 -> Switch1/3
  Add/1 -> EtherCAT PDO Transmit02/1
  Bus Selector/3 -> Switch1/2  "<SenseMinusBroken>"
  Switch1/1 -> Add/3
  Bus Selector/1 -> Range Assert/1(u)  "<FaultState>"

== system sgMdl_BMTS_FaultInsertionWithFIU/BMTS Write /Subsystem/FIU_Ch_09 ==
  note: Update
  Data : Inport  OutDataTypeStr=Bus: FIU_Set
  Add : Sum  Inputs=+++
  Bus Selector : BusSelector  OutputSignals=FaultState,SensePlusBroken,SenseMinusBroken
  Constant3 : Constant  Value=8  OutDataTypeStr=uint8
  Constant4 : Constant  Value=0  OutDataTypeStr=uint8
  Constant6 : Constant  Value=16  OutDataTypeStr=uint8
  Constant7 : Constant  Value=0  OutDataTypeStr=uint8
  EtherCAT PDO Transmit02 : slrealtimeethercatlib/EtherCAT PDO Transmit  Priority=3  sig_name=Device_01 (FIU12).Rx_Channel_09.faultState  sig_offset=64  sig_type=uint8  type_size=8  sig_dim=1  device_id=1  sample_time=0.001000
  Range Assert : MATLAB Function  TreatAsAtomicUnit=on
  Switch : Switch  Criteria=u2 > Threshold  SaturateOnIntegerOverflow=off  InputSameDT=off
  Switch1 : Switch  Criteria=u2 > Threshold  SaturateOnIntegerOverflow=off  InputSameDT=off
  wires:
  Range Assert/1(y) -> Add/1
  Data/1 -> Bus Selector/1
  Bus Selector/2 -> Switch/2  "<SensePlusBroken>"
  Constant6/1 -> Switch1/1
  Constant3/1 -> Switch/1
  Switch/1 -> Add/2
  Constant4/1 -> Switch/3
  Constant7/1 -> Switch1/3
  Add/1 -> EtherCAT PDO Transmit02/1
  Bus Selector/3 -> Switch1/2  "<SenseMinusBroken>"
  Switch1/1 -> Add/3
  Bus Selector/1 -> Range Assert/1(u)  "<FaultState>"

== system sgMdl_BMTS_FaultInsertionWithFIU/BMTS Write /Subsystem/FIU_Ch_10 ==
  note: Update
  Data : Inport  OutDataTypeStr=Bus: FIU_Set
  Add : Sum  Inputs=+++
  Bus Selector : BusSelector  OutputSignals=FaultState,SensePlusBroken,SenseMinusBroken
  Constant3 : Constant  Value=8  OutDataTypeStr=uint8
  Constant4 : Constant  Value=0  OutDataTypeStr=uint8
  Constant6 : Constant  Value=16  OutDataTypeStr=uint8
  Constant7 : Constant  Value=0  OutDataTypeStr=uint8
  EtherCAT PDO Transmit02 : slrealtimeethercatlib/EtherCAT PDO Transmit  Priority=3  sig_name=Device_01 (FIU12).Rx_Channel_10.faultState  sig_offset=72  sig_type=uint8  type_size=8  sig_dim=1  device_id=1  sample_time=0.001000
  Range Assert : MATLAB Function  TreatAsAtomicUnit=on
  Switch : Switch  Criteria=u2 > Threshold  SaturateOnIntegerOverflow=off  InputSameDT=off
  Switch1 : Switch  Criteria=u2 > Threshold  SaturateOnIntegerOverflow=off  InputSameDT=off
  wires:
  Range Assert/1(y) -> Add/1
  Data/1 -> Bus Selector/1
  Bus Selector/2 -> Switch/2  "<SensePlusBroken>"
  Constant6/1 -> Switch1/1
  Constant3/1 -> Switch/1
  Switch/1 -> Add/2
  Constant4/1 -> Switch/3
  Constant7/1 -> Switch1/3
  Add/1 -> EtherCAT PDO Transmit02/1
  Bus Selector/3 -> Switch1/2  "<SenseMinusBroken>"
  Switch1/1 -> Add/3
  Bus Selector/1 -> Range Assert/1(u)  "<FaultState>"

== system sgMdl_BMTS_FaultInsertionWithFIU/BMTS Write /Subsystem/FIU_Ch_11 ==
  note: Update
  Data : Inport  OutDataTypeStr=Bus: FIU_Set
  Add : Sum  Inputs=+++
  Bus Selector : BusSelector  OutputSignals=FaultState,SensePlusBroken,SenseMinusBroken
  Constant3 : Constant  Value=8  OutDataTypeStr=uint8
  Constant4 : Constant  Value=0  OutDataTypeStr=uint8
  Constant6 : Constant  Value=16  OutDataTypeStr=uint8
  Constant7 : Constant  Value=0  OutDataTypeStr=uint8
  EtherCAT PDO Transmit02 : slrealtimeethercatlib/EtherCAT PDO Transmit  Priority=3  sig_name=Device_01 (FIU12).Rx_Channel_11.faultState  sig_offset=80  sig_type=uint8  type_size=8  sig_dim=1  device_id=1  sample_time=0.001000
  Range Assert : MATLAB Function  TreatAsAtomicUnit=on
  Switch : Switch  Criteria=u2 > Threshold  SaturateOnIntegerOverflow=off  InputSameDT=off
  Switch1 : Switch  Criteria=u2 > Threshold  SaturateOnIntegerOverflow=off  InputSameDT=off
  wires:
  Range Assert/1(y) -> Add/1
  Data/1 -> Bus Selector/1
  Bus Selector/2 -> Switch/2  "<SensePlusBroken>"
  Constant6/1 -> Switch1/1
  Constant3/1 -> Switch/1
  Switch/1 -> Add/2
  Constant4/1 -> Switch/3
  Constant7/1 -> Switch1/3
  Add/1 -> EtherCAT PDO Transmit02/1
  Bus Selector/3 -> Switch1/2  "<SenseMinusBroken>"
  Switch1/1 -> Add/3
  Bus Selector/1 -> Range Assert/1(u)  "<FaultState>"

== system sgMdl_BMTS_FaultInsertionWithFIU/BMTS Write /Subsystem/FIU_Ch_12 ==
  note: Update
  Data : Inport  OutDataTypeStr=Bus: FIU_Set
  Add : Sum  Inputs=+++
  Bus Selector : BusSelector  OutputSignals=FaultState,SensePlusBroken,SenseMinusBroken
  Constant3 : Constant  Value=8  OutDataTypeStr=uint8
  Constant4 : Constant  Value=0  OutDataTypeStr=uint8
  Constant6 : Constant  Value=16  OutDataTypeStr=uint8
  Constant7 : Constant  Value=0  OutDataTypeStr=uint8
  EtherCAT PDO Transmit02 : slrealtimeethercatlib/EtherCAT PDO Transmit  Priority=3  sig_name=Device_01 (FIU12).Rx_Channel_12.faultState  sig_offset=88  sig_type=uint8  type_size=8  sig_dim=1  device_id=1  sample_time=0.001000
  Range Assert : MATLAB Function  TreatAsAtomicUnit=on
  Switch : Switch  Criteria=u2 > Threshold  SaturateOnIntegerOverflow=off  InputSameDT=off
  Switch1 : Switch  Criteria=u2 > Threshold  SaturateOnIntegerOverflow=off  InputSameDT=off
  wires:
  Range Assert/1(y) -> Add/1
  Data/1 -> Bus Selector/1
  Bus Selector/2 -> Switch/2  "<SensePlusBroken>"
  Constant6/1 -> Switch1/1
  Constant3/1 -> Switch/1
  Switch/1 -> Add/2
  Constant4/1 -> Switch/3
  Constant7/1 -> Switch1/3
  Add/1 -> EtherCAT PDO Transmit02/1
  Bus Selector/3 -> Switch1/2  "<SenseMinusBroken>"
  Switch1/1 -> Add/3
  Bus Selector/1 -> Range Assert/1(u)  "<FaultState>"

== system sgMdl_BMTS_FaultInsertionWithFIU/BMTS Write /Subsystem/FIU_Ch_01/EtherCAT State Control ==
  EC OP State : Constant  Value=8  OutDataTypeStr=int32
  EC State Compare : simulink/Logic and Bit Operations/Compare To Constant  relop=~=  const=8  OutDataTypeStr=boolean
  Get SubDevice State : slrealtimeethercatlib/Get SubDevice State  device_id=1  subdevice_name=Device_01 (FIU12)  sample_time=0.001  subdevice_addr=1001  selected_subdevice=Term 1 (EK1100)  timeout=500  subdevice_found=1
  Set SubDevice State : slrealtimeethercatlib/Set SubDevice State  device_id=1  subdevice_name=Device_01 (FIU12)  sample_time=0.001  subdevice_addr=1001  selected_subdevice=Term 1 (EK1100)  subdevice_found=1
  Terminator1 : Terminator
  Terminator2 : Terminator
  wires:
  EC OP State/1 -> Set SubDevice State/1
  Get SubDevice State/1 -> EC State Compare/1
  Set SubDevice State/1 -> Terminator1/1
  EC State Compare/1 -> Set SubDevice State/2
  Set SubDevice State/2 -> Terminator2/1

== matlab function sgMdl_BMTS_FaultInsertionWithFIU/BMTS Write /Subsystem/FIU_Ch_02/Range Assert ==
  data: u input; y output
function y = fcn(u)

    y = sg_bce.fiuFaultStateRangeAssert(u);

end

== matlab function sgMdl_BMTS_FaultInsertionWithFIU/BMTS Write /Subsystem/FIU_Ch_03/Range Assert ==
  data: u input; y output
function y = fcn(u)

    y = sg_bce.fiuFaultStateRangeAssert(u);

end

== matlab function sgMdl_BMTS_FaultInsertionWithFIU/BMTS Write /Subsystem/FIU_Ch_04/Range Assert ==
  data: u input; y output
function y = fcn(u)

    y = sg_bce.fiuFaultStateRangeAssert(u);

end

== matlab function sgMdl_BMTS_FaultInsertionWithFIU/BMTS Write /Subsystem/FIU_Ch_05/Range Assert ==
  data: u input; y output
function y = fcn(u)

    y = sg_bce.fiuFaultStateRangeAssert(u);

end

== matlab function sgMdl_BMTS_FaultInsertionWithFIU/BMTS Write /Subsystem/FIU_Ch_06/Range Assert ==
  data: u input; y output
function y = fcn(u)

    y = sg_bce.fiuFaultStateRangeAssert(u);

end

== matlab function sgMdl_BMTS_FaultInsertionWithFIU/BMTS Write /Subsystem/FIU_Ch_07/Range Assert ==
  data: u input; y output
function y = fcn(u)

    y = sg_bce.fiuFaultStateRangeAssert(u);

end

== matlab function sgMdl_BMTS_FaultInsertionWithFIU/BMTS Write /Subsystem/FIU_Ch_08/Range Assert ==
  data: u input; y output
function y = fcn(u)

    y = sg_bce.fiuFaultStateRangeAssert(u);

end

== matlab function sgMdl_BMTS_FaultInsertionWithFIU/BMTS Write /Subsystem/FIU_Ch_09/Range Assert ==
  data: u input; y output
function y = fcn(u)

    y = sg_bce.fiuFaultStateRangeAssert(u);

end

== matlab function sgMdl_BMTS_FaultInsertionWithFIU/BMTS Write /Subsystem/FIU_Ch_01/Range Assert ==
  data: u input; y output
function y = fcn(u)

    y = sg_bce.fiuFaultStateRangeAssert(u);

end

== matlab function sgMdl_BMTS_FaultInsertionWithFIU/BMTS Write /Subsystem/FIU_Ch_10/Range Assert ==
  data: u input; y output
function y = fcn(u)

    y = sg_bce.fiuFaultStateRangeAssert(u);

end

== matlab function sgMdl_BMTS_FaultInsertionWithFIU/BMTS Write /Subsystem/FIU_Ch_11/Range Assert ==
  data: u input; y output
function y = fcn(u)

    y = sg_bce.fiuFaultStateRangeAssert(u);

end

== matlab function sgMdl_BMTS_FaultInsertionWithFIU/BMTS Write /Subsystem/FIU_Ch_12/Range Assert ==
  data: u input; y output
function y = fcn(u)

    y = sg_bce.fiuFaultStateRangeAssert(u);

end
